simulink model "sim_RCclen"  (Simulink 7.5)
settings: Solver=ode45  StartTime=0.0  StopTime=8000  RelTol=1e-3
settings Model: Creator=Jaroslav Fait  LastModifiedBy=Jaroslav Fait  ExtModeTrigMode=oneshot  ExtModeArmWhenConnect=off
settings DataIOCC: LimitDataPoints=off
settings OptimizationCC: BlockReduction=off  BooleanDataType=off
settings DebuggingCC: SaveWithParameterizedLinksMsg=none  SignalResolutionControl=TryResolveAllWithWarning  SolverPrmCheckMsg=none  MultiTaskDSMMsg=warning  MultiTaskCondExecSysMsg=none  StrictBusMsg=None
settings HardwareCC: TargetUnknown=on
settings RTWCC: IncludeERTFirstTime=on

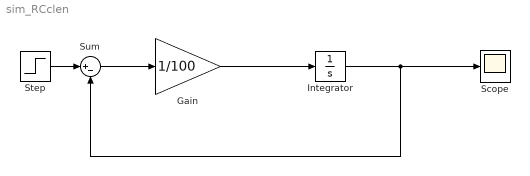
== system sim_RCclen ==
  Gain : Gain  Gain=1/100  SaturateOnIntegerOverflow=on  OutDataTypeStr=Inherit: Same as input  ParamDataTypeStr=Inherit: Same as input
  Integrator : Integrator
  Scope : Scope
  Step : Step  Time=0  After=220  SampleTime=0
  Sum : Sum  Inputs=|+-  SaturateOnIntegerOverflow=on  InputSameDT=on  OutDataTypeStr=Inherit: Same as first input
  wires:
  Sum/1 -> Gain/1
  Step/1 -> Sum/1
  Gain/1 -> Integrator/1
  Integrator/1 -> Sum/2, Scope/1
